simulink model "SAR_model"  (R2022a)
settings: Solver=VariableStepAuto  StartTime=0.0  StopTime=100  FixedStep=5
values from neighbouring files (symbols this model uses):
  C = diag([0.1789, 0.3915,  0.3126, 0.1245])    [Initialization.m]
  delta = 0.5*[ 1.3523 1.2784 2.1553 ... (first row only)    [Initialization.m]
  eta0 = [0 0 0 0]    [Initialization.m]
  J = [10 1 1; 1 8 0; 1 0 6]    [Initialization.m]
  K = diag([2.5514, 5.1806, 3.8173, 6.1966])    [Initialization.m]
  psi0 = delta*transpose(w0)    [Initialization.m]
  q0 = angle2quat(Phi0(1),Phi0(2),Phi0(3))    [Initialization.m]
  qd = angle2quat(Phid(1),Phid(2),Phid(3))    [Initialization.m]
  w0 = [pi/12 pi/24 0]    [Initialization.m]
  wd = [0 0 0]    [Initialization.m]
undefined symbols (not defined in the file or in its folder): deg, magnitude, rad, s
libraries: aerolibconvert2 x3, sharedtransform x2, rllib x2, aerolibutil x1
settings Model: PacingRate=1000  Creator=Ali  LastModifiedBy=Shayan
settings SolverCC: MaxConsecutiveZCs=1  MaxConsecutiveMinStep=10  ZeroCrossAlgorithm=Adaptive  AlgebraicLoopSolver=TrustRegion
settings DataIOCC: SaveFinalState=on  SaveState=on  LoggingToFile=on
settings DebuggingCC: AlgebraicLoopMsg=none  UnconnectedInputMsg=warning  UnconnectedOutputMsg=warning  UnconnectedLineMsg=warning  SFMachineParentedDataDiag=warning
settings ModelReferenceCC: ModelReferenceMinAlgLoopOccurrences=on

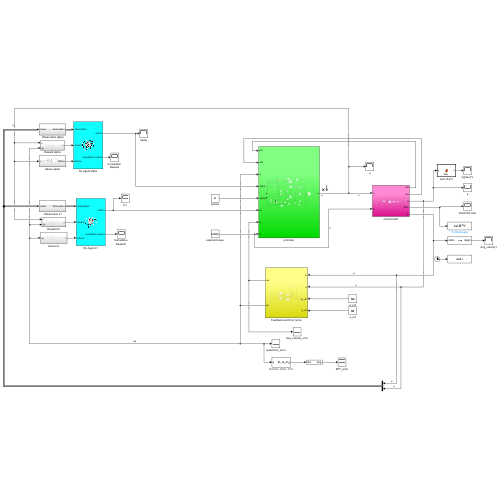
[thumbnail: Simulink's stored preview of the top-level diagram]
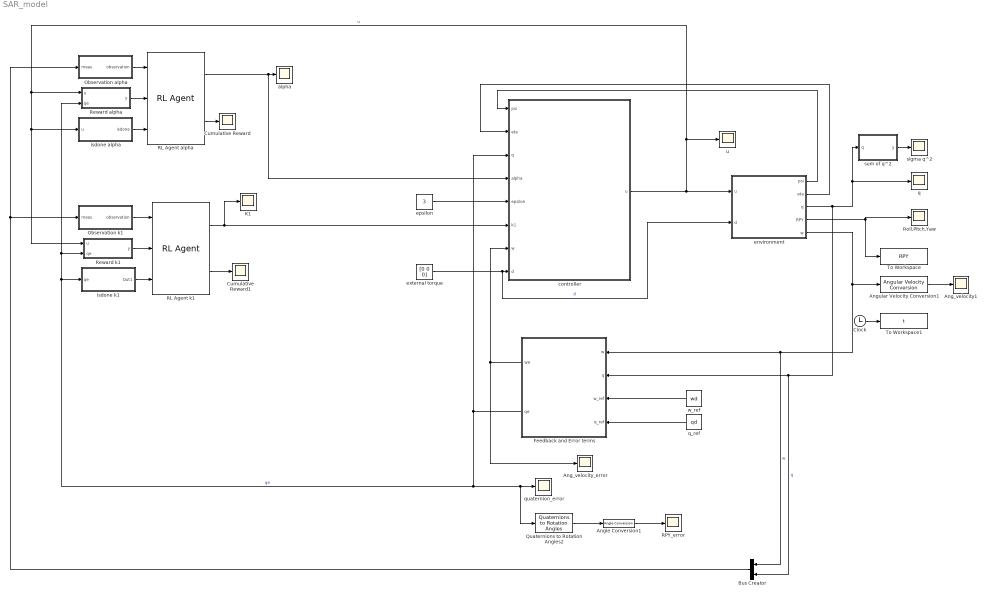
== system SAR_model ==
  " Observation alpha" : Subsystem
  " Observation k1" : Subsystem
  Ang_velocity1 : Scope
  Ang_velocity_error : Scope
  Angle Conversion1 : aerolibconvert2/Angle Conversion  IU=rad  OU=deg
  Angular Velocity Conversion1 : aerolibconvert2/Angular Velocity Conversion  IU=rad/s  OU=deg/s
  Bus Creator : BusCreator  Inputs=2
  Clock : Clock
  Cumulative Reward : Scope
  Cumulative Reward1 : Scope
  Feedback and Error terms : Subsystem
  K1 : Scope
  Quaternions to Rotation Angles2 : sharedtransform/Quaternions to Rotation Angles  rotationOrder=ZYX  aMode=aMode
      settings: SourceProductBaseCode=AE,PW,DR,MT,VE
  RL Agent alpha : rllib/RL Agent  Agent=agent3_Trained  ExternalActionAsInput=off  ProvideLastAction=off  ProvideCumRwd=on  TreatAsDirectFeedthrough=on  UseStrictObservationDataTypes=off
      settings: SourceProductName=Reinforcement Learning
  RL Agent k1 : rllib/RL Agent  Agent=agent1  ExternalActionAsInput=off  ProvideLastAction=off  ProvideCumRwd=on  TreatAsDirectFeedthrough=on  UseStrictObservationDataTypes=off
      settings: SourceProductName=Reinforcement Learning
  RPY_error : Scope
  Reward alpha : Subsystem
  Reward k1 : Subsystem
  Roll,Pitch,Yaw : Scope
  To Workspace : ToWorkspace  VariableName=RPY  SaveFormat=Timeseries
  To Workspace1 : ToWorkspace  VariableName=t  SaveFormat=Timeseries
  alpha : Scope
  "controller " : Subsystem
  environment : Subsystem
  epsilon : Constant  Value=3
  external torque : Constant  Value=[0 0 0]
  isdone alpha : Subsystem
  isdone k1 : Subsystem
  q : Scope
  q_ref : Constant  Value=qd
  quaternion_error : Scope
  sigma q^2 : Scope
  sum of q^2 : MATLAB Function  TreatAsAtomicUnit=on
  u : Scope
  w_ref : Constant  Value=wd
  wires:
  epsilon/1 -> "controller "/5(epsilon)
  external torque/1 -> environment/2(d), "controller "/8(d)  "d"
  Feedback and Error terms/1(we) -> Ang_velocity_error/1, "controller "/7(w)
  w_ref/1 -> Feedback and Error terms/3(w_ref)
  q_ref/1 -> Feedback and Error terms/4(q_ref)
  Quaternions to Rotation Angles2/1 -> Angle Conversion1/1
  Angle Conversion1/1 -> RPY_error/1
  isdone alpha/1(isdone) -> RL Agent alpha/3
  Reward alpha/1(y) -> RL Agent alpha/2
  RL Agent alpha/2 -> Cumulative Reward/1
  " Observation alpha"/1(observation) -> RL Agent alpha/1
  "controller "/1(u) -> environment/1(u), Reward alpha/1(u), isdone alpha/1(u), Reward k1/1(u), u/1  "u"
  RL Agent k1/2 -> Cumulative Reward1/1
  Bus Creator/1 -> " Observation alpha"/1(meas), " Observation k1"/1(meas)
  Reward k1/1(y) -> RL Agent k1/2
  " Observation k1"/1(observation) -> RL Agent k1/1
  Feedback and Error terms/2(qe) -> quaternion_error/1, Quaternions to Rotation Angles2/1, Reward alpha/2(qe), Reward k1/2(qe), isdone k1/1(qe), "controller "/3(q)  "qe"
  RL Agent alpha/1 -> "controller "/4(alpha), alpha/1
  isdone k1/1(Out1) -> RL Agent k1/3
  Clock/1 -> To Workspace1/1
  RL Agent k1/1 -> K1/1, "controller "/6(k1)
  sum of q^2/1(y) -> sigma q^2/1
  environment/3(q) -> sum of q^2/1(q), q/1, Feedback and Error terms/2(q), Bus Creator/2  "q"
  environment/4(RPY) -> To Workspace/1, Roll,Pitch,Yaw/1
  environment/5(w) -> Feedback and Error terms/1(w), Bus Creator/1, Angular Velocity Conversion1/1  "w"
  environment/1(psi) -> "controller "/1(psi)
  environment/2(eta) -> "controller "/2(eta)
  Angular Velocity Conversion1/1 -> Ang_velocity1/1

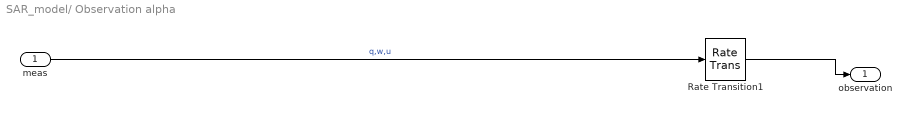
== system SAR_model/ Observation alpha ==
  meas : Inport
  Rate Transition1 : RateTransition
  observation : Outport  VectorParamsAs1DForOutWhenUnconnected=off
  wires:
  meas/1 -> Rate Transition1/1  "q,w,u"
  Rate Transition1/1 -> observation/1

== system SAR_model/ Observation k1 ==
  meas : Inport
  Rate Transition1 : RateTransition
  observation : Outport  VectorParamsAs1DForOutWhenUnconnected=off
  wires:
  meas/1 -> Rate Transition1/1  "q,w,u"
  Rate Transition1/1 -> observation/1

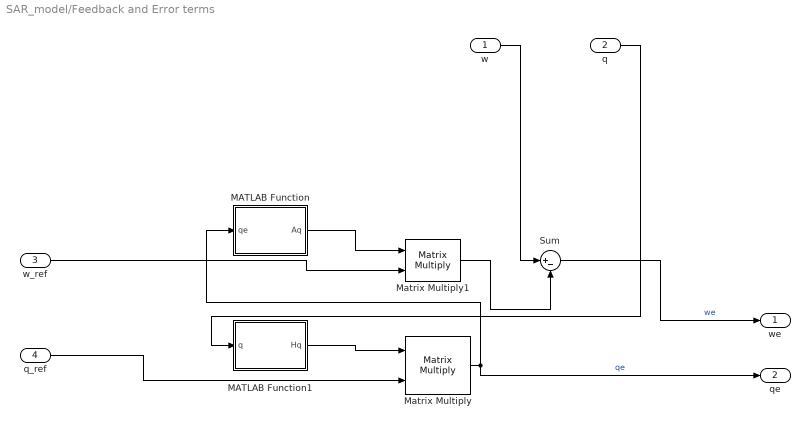
== system SAR_model/Feedback and Error terms ==
  w : Inport
  q : Inport  Port=2
  w_ref : Inport  Port=3
  q_ref : Inport  Port=4
  MATLAB Function : MATLAB Function  TreatAsAtomicUnit=on
  MATLAB Function1 : MATLAB Function  TreatAsAtomicUnit=on
  Matrix Multiply : Product  Multiplication=Matrix(*)
  Matrix Multiply1 : Product  Multiplication=Matrix(*)
  Sum : Sum  Inputs=|+-
  we : Outport
  qe : Outport  Port=2
  wires:
  Sum/1 -> we/1  "we"
  MATLAB Function1/1(Hq) -> Matrix Multiply/1
  Matrix Multiply1/1 -> Sum/2
  Matrix Multiply/1 -> qe/1, MATLAB Function/1(qe)  "qe"
  w/1 -> Sum/1
  q_ref/1 -> Matrix Multiply/2
  q/1 -> MATLAB Function1/1(q)
  w_ref/1 -> Matrix Multiply1/2
  MATLAB Function/1(Aq) -> Matrix Multiply1/1

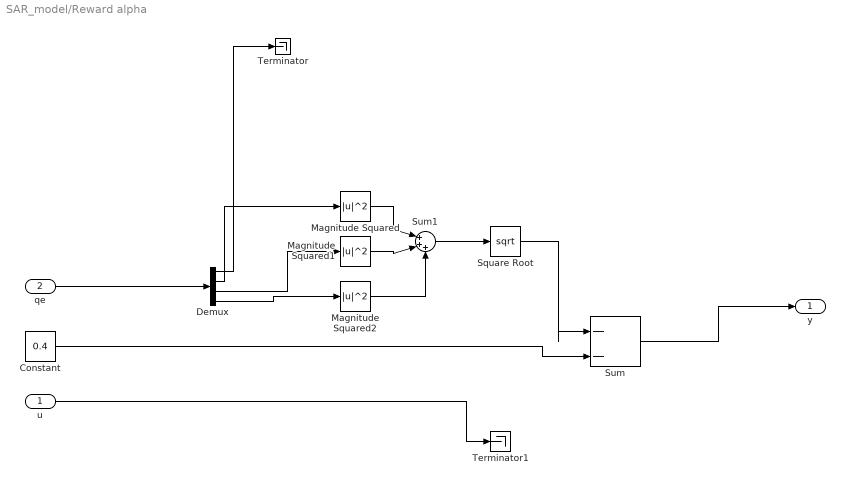
== system SAR_model/Reward alpha ==
  u : Inport
  qe : Inport  Port=2
  Constant : Constant  Value=0.4
  Demux : Demux
  Magnitude Squared : Math  Operator=magnitude^2
  Magnitude Squared1 : Math  Operator=magnitude^2
  Magnitude Squared2 : Math  Operator=magnitude^2
  Square Root : Sqrt
  Sum : Sum  Inputs=|--
  Sum1 : Sum  Inputs=|+++
  Terminator : Terminator
  Terminator1 : Terminator
  y : Outport
  wires:
  u/1 -> Terminator1/1
  Constant/1 -> Sum/2
  Sum/1 -> y/1
  qe/1 -> Demux/1
  Demux/1 -> Terminator/1
  Demux/2 -> Magnitude Squared/1
  Demux/3 -> Magnitude Squared1/1
  Demux/4 -> Magnitude Squared2/1
  Magnitude Squared/1 -> Sum1/1
  Magnitude Squared1/1 -> Sum1/2
  Magnitude Squared2/1 -> Sum1/3
  Sum1/1 -> Square Root/1
  Square Root/1 -> Sum/1

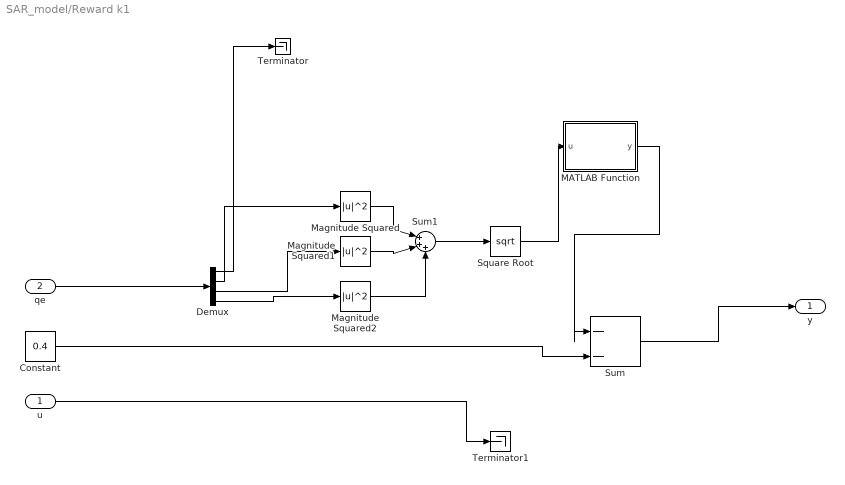
== system SAR_model/Reward k1 ==
  u : Inport
  qe : Inport  Port=2
  Constant : Constant  Value=0.4
  Demux : Demux
  MATLAB Function : MATLAB Function  TreatAsAtomicUnit=on
  Magnitude Squared : Math  Operator=magnitude^2
  Magnitude Squared1 : Math  Operator=magnitude^2
  Magnitude Squared2 : Math  Operator=magnitude^2
  Square Root : Sqrt
  Sum : Sum  Inputs=|--
  Sum1 : Sum  Inputs=|+++
  Terminator : Terminator
  Terminator1 : Terminator
  y : Outport
  wires:
  u/1 -> Terminator1/1
  Constant/1 -> Sum/2
  Sum/1 -> y/1
  qe/1 -> Demux/1
  Demux/1 -> Terminator/1
  Demux/2 -> Magnitude Squared/1
  Demux/3 -> Magnitude Squared1/1
  Demux/4 -> Magnitude Squared2/1
  Magnitude Squared/1 -> Sum1/1
  Magnitude Squared1/1 -> Sum1/2
  Magnitude Squared2/1 -> Sum1/3
  Sum1/1 -> Square Root/1
  Square Root/1 -> MATLAB Function/1(u)
  MATLAB Function/1(y) -> Sum/1

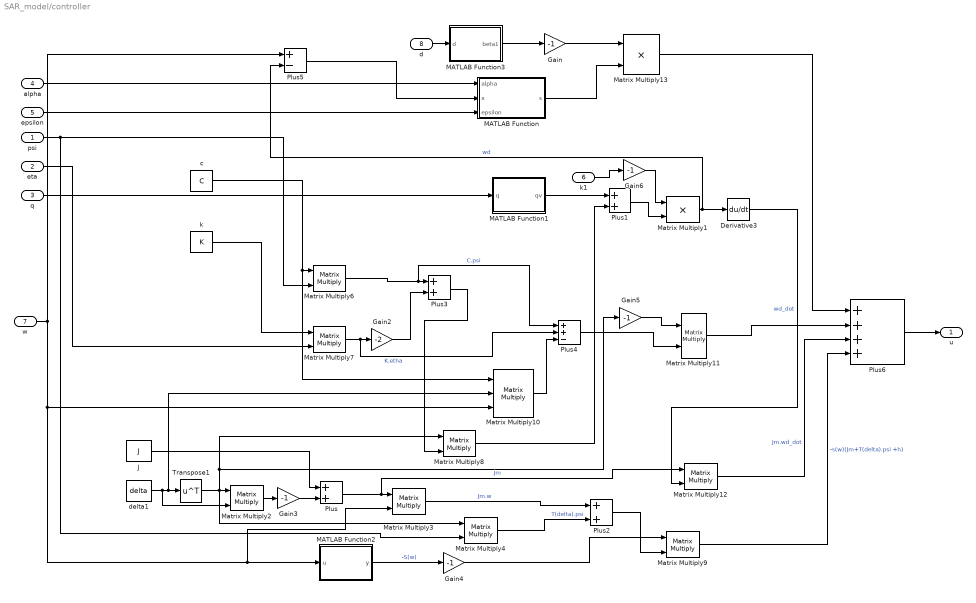
== system SAR_model/controller  ==
  psi : Inport
  eta : Inport  Port=2
  q : Inport  Port=3
  alpha : Inport  Port=4
  epsilon : Inport  Port=5
  k1 : Inport  Port=6
  w : Inport  Port=7
  d : Inport  Port=8
  Derivative3 : Derivative
  Gain{,3..6} (5 alike) : Gain  Gain=-1
  Gain2 : Gain  Gain=-2
  J : Constant  Value=J
  MATLAB Function : MATLAB Function  TreatAsAtomicUnit=on
  MATLAB Function1 : MATLAB Function  TreatAsAtomicUnit=on
  MATLAB Function2 : MATLAB Function  TreatAsAtomicUnit=on
  MATLAB Function3 : MATLAB Function  TreatAsAtomicUnit=on
  Matrix Multiply1 : Product
  Matrix Multiply10 : Product  Inputs=3  Multiplication=Matrix(*)
  Matrix Multiply{2..4,7..9,11..12} (8 alike) : Product  Multiplication=Matrix(*)
  Matrix Multiply13 : Product
  Matrix Multiply6 : Product  Multiplication=Matrix(*)  InputSameDT=on
  Plus{,1..3} (4 alike) : Sum
  Plus4 : Sum  Inputs=++-
  Plus5 : Sum  Inputs=+-
  Plus6 : Sum  Inputs=++++
  Transpose1 : Math  Operator=transpose
  c : Constant  Value=C
  delta1 : Constant  Value=delta
  k : Constant  Value=K
  u : Outport
  wires:
  Matrix Multiply6/1 -> Plus4/1, Plus3/1  "C.psi"
  Matrix Multiply7/1 -> Plus4/2, Gain2/1  "K.etha"
  Gain2/1 -> Plus3/2
  Plus3/1 -> Matrix Multiply8/2
  alpha/1 -> MATLAB Function/1(alpha)
  epsilon/1 -> MATLAB Function/3(epsilon)
  q/1 -> MATLAB Function1/1(q)
  Matrix Multiply8/1 -> Plus1/2
  MATLAB Function1/1(qv) -> Plus1/1
  k1/1 -> Gain6/1
  Matrix Multiply1/1 -> Derivative3/1, Plus5/2  "wd"
  psi/1 -> Matrix Multiply6/2, Matrix Multiply4/2
  eta/1 -> Matrix Multiply7/2
  delta1/1 -> Matrix Multiply2/2, Matrix Multiply10/2, Transpose1/1
  Plus/1 -> Matrix Multiply12/1, Matrix Multiply3/1  "Jm"
  J/1 -> Plus/1
  Gain3/1 -> Plus/2
  Matrix Multiply2/1 -> Gain3/1
  Transpose1/1 -> Matrix Multiply8/1, Gain5/1, Matrix Multiply2/1, Matrix Multiply4/1
  w/1 -> Plus5/1, Matrix Multiply10/3, Matrix Multiply3/2, MATLAB Function2/1(u)
  MATLAB Function2/1(y) -> Gain4/1  "-S(w)"
  Matrix Multiply3/1 -> Plus2/1  "Jm.w"
  Matrix Multiply4/1 -> Plus2/2  "T(delta).psi"
  Plus2/1 -> Matrix Multiply9/2
  Matrix Multiply10/1 -> Plus4/3
  Plus4/1 -> Matrix Multiply11/2
  Gain5/1 -> Matrix Multiply11/1
  d/1 -> MATLAB Function3/1(d)
  Plus5/1 -> MATLAB Function/2(x)
  Matrix Multiply9/1 -> Plus6/4  "-s(w)(Jm+T(delta).psi +h)"
  Matrix Multiply11/1 -> Plus6/2
  Matrix Multiply12/1 -> Plus6/3  "Jm.wd_dot"
  Matrix Multiply13/1 -> Plus6/1
  Plus6/1 -> u/1
  Derivative3/1 -> Matrix Multiply12/2  "wd_dot"
  c/1 -> Matrix Multiply10/1, Matrix Multiply6/1
  k/1 -> Matrix Multiply7/1
  Plus1/1 -> Matrix Multiply1/2
  Gain6/1 -> Matrix Multiply1/1
  MATLAB Function/1(s) -> Matrix Multiply13/2
  MATLAB Function3/1(beta1) -> Gain/1
  Gain/1 -> Matrix Multiply13/1
  Gain4/1 -> Matrix Multiply9/1

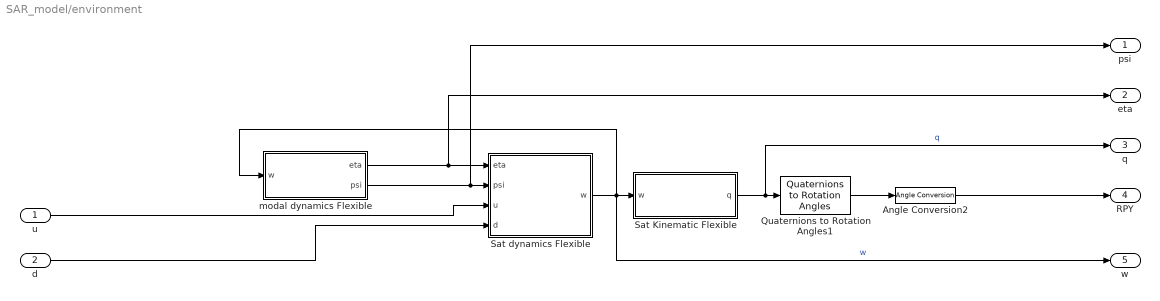
== system SAR_model/environment ==
  u : Inport
  d : Inport  Port=2
  Angle Conversion2 : aerolibconvert2/Angle Conversion  IU=rad  OU=deg
  Quaternions to Rotation Angles1 : sharedtransform/Quaternions to Rotation Angles  rotationOrder=ZYX  aMode=aMode
      settings: SourceProductBaseCode=AE,PW,DR,MT,VE
  Sat Kinematic Flexible : Subsystem
  Sat dynamics Flexible : Subsystem
  modal dynamics Flexible : Subsystem
  psi : Outport
  eta : Outport  Port=2
  q : Outport  Port=3
  RPY : Outport  Port=4
  w : Outport  Port=5
  wires:
  Sat dynamics Flexible/1(w) -> w/1, modal dynamics Flexible/1(w), Sat Kinematic Flexible/1(w)  "w"
  modal dynamics Flexible/1(eta) -> Sat dynamics Flexible/1(eta), eta/1
  modal dynamics Flexible/2(psi) -> Sat dynamics Flexible/2(psi), psi/1
  u/1 -> Sat dynamics Flexible/3(u)
  d/1 -> Sat dynamics Flexible/4(d)
  Sat Kinematic Flexible/1(q) -> q/1, Quaternions to Rotation Angles1/1  "q"
  Quaternions to Rotation Angles1/1 -> Angle Conversion2/1
  Angle Conversion2/1 -> RPY/1

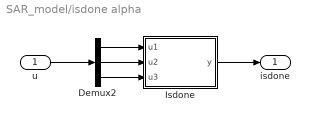
== system SAR_model/isdone alpha ==
  u : Inport
  Demux2 : Demux  Outputs=3
  "Isdone " : MATLAB Function  TreatAsAtomicUnit=on
  isdone : Outport
  wires:
  u/1 -> Demux2/1
  Demux2/1 -> "Isdone "/1(u1)
  Demux2/2 -> "Isdone "/2(u2)
  Demux2/3 -> "Isdone "/3(u3)
  "Isdone "/1(y) -> isdone/1

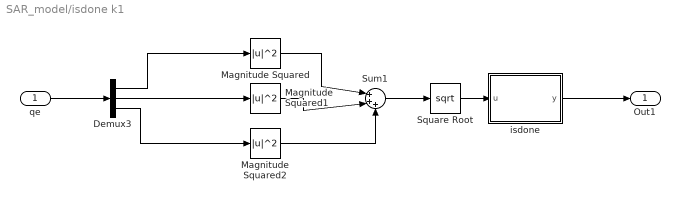
== system SAR_model/isdone k1 ==
  qe : Inport
  Demux3 : Demux  Outputs=3
  Magnitude Squared : Math  Operator=magnitude^2
  Magnitude Squared1 : Math  Operator=magnitude^2
  Magnitude Squared2 : Math  Operator=magnitude^2
  Square Root : Sqrt
  Sum1 : Sum  Inputs=|+++
  isdone : MATLAB Function  TreatAsAtomicUnit=on
  Out1 : Outport
  wires:
  Square Root/1 -> isdone/1(u)
  Magnitude Squared/1 -> Sum1/1
  Demux3/2 -> Magnitude Squared1/1
  Magnitude Squared2/1 -> Sum1/3
  Magnitude Squared1/1 -> Sum1/2
  Demux3/1 -> Magnitude Squared/1
  Sum1/1 -> Square Root/1
  Demux3/3 -> Magnitude Squared2/1
  qe/1 -> Demux3/1
  isdone/1(y) -> Out1/1

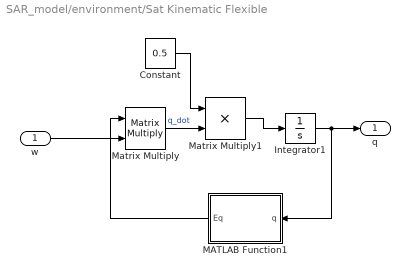
== system SAR_model/environment/Sat Kinematic Flexible ==
  w : Inport
  Constant : Constant  Value=0.5
  Integrator1 : Integrator  InitialCondition=q0  ContinuousStateAttributes='q'
  MATLAB Function1 : MATLAB Function  TreatAsAtomicUnit=on
  Matrix Multiply : Product  Multiplication=Matrix(*)
  Matrix Multiply1 : Product
  q : Outport
  wires:
  Matrix Multiply/1 -> Matrix Multiply1/2  "q_dot"
  w/1 -> Matrix Multiply/2
  Integrator1/1 -> MATLAB Function1/1(q), q/1
  MATLAB Function1/1(Eq) -> Matrix Multiply/1
  Matrix Multiply1/1 -> Integrator1/1
  Constant/1 -> Matrix Multiply1/1

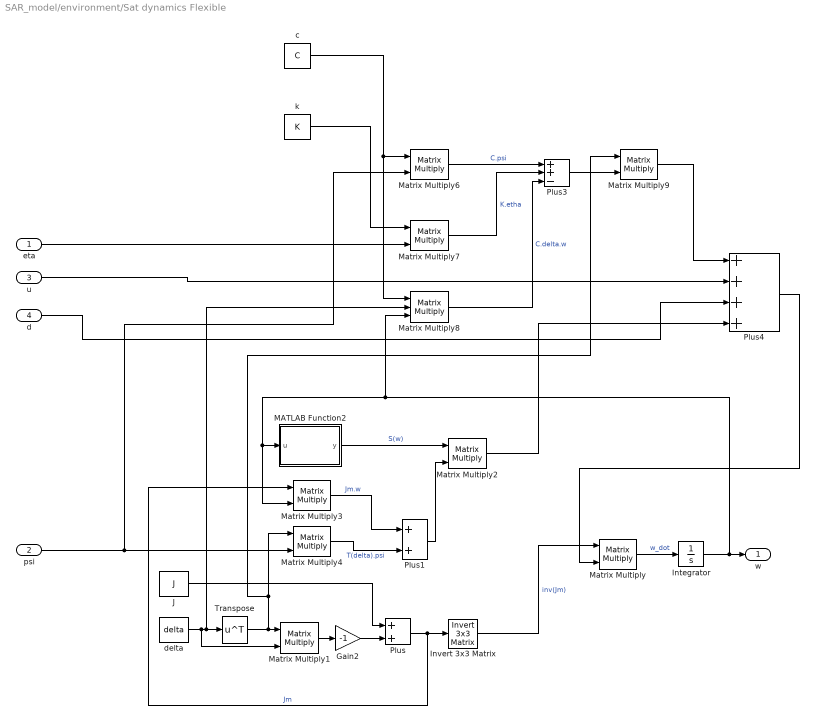
== system SAR_model/environment/Sat dynamics Flexible ==
  eta : Inport
  psi : Inport  Port=2
  u : Inport  Port=3
  d : Inport  Port=4
  Gain2 : Gain  Gain=-1
  Integrator : Integrator  InitialCondition=w0  ContinuousStateAttributes='w'
  Invert 3x3 Matrix : aerolibutil/Invert  3x3 Matrix
  J : Constant  Value=J
  MATLAB Function2 : MATLAB Function  TreatAsAtomicUnit=on
  Matrix Multiply{,1..4,7} (6 alike) : Product  Multiplication=Matrix(*)
  Matrix Multiply6 : Product  Multiplication=Matrix(*)  InputSameDT=on
  Matrix Multiply8 : Product  Inputs=3  Multiplication=Matrix(*)
  Matrix Multiply9 : Product  Multiplication=Matrix(*)  InputSameDT=on
  Plus : Sum
  Plus1 : Sum
  Plus3 : Sum  Inputs=++-
  Plus4 : Sum  Inputs=++++
  Transpose : Math  Operator=transpose
  c : Constant  Value=C  VectorParams1D=off
  delta : Constant  Value=delta
  k : Constant  Value=K  VectorParams1D=off
  w : Outport
  wires:
  Integrator/1 -> Matrix Multiply8/3, Matrix Multiply3/2, MATLAB Function2/1(u), w/1
  delta/1 -> Matrix Multiply1/2, Matrix Multiply8/2, Transpose/1
  Transpose/1 -> Matrix Multiply9/1, Matrix Multiply4/1, Matrix Multiply1/1
  Matrix Multiply1/1 -> Gain2/1
  Gain2/1 -> Plus/2
  J/1 -> Plus/1
  Plus/1 -> Invert 3x3 Matrix/1, Matrix Multiply3/1  "Jm"
  Invert 3x3 Matrix/1 -> Matrix Multiply/1  "inv(Jm)"
  MATLAB Function2/1(y) -> Matrix Multiply2/1  "S(w)"
  psi/1 -> Matrix Multiply6/2, Matrix Multiply4/2
  Matrix Multiply3/1 -> Plus1/1  "Jm.w"
  Matrix Multiply4/1 -> Plus1/2  "T(delta).psi"
  Plus1/1 -> Matrix Multiply2/2
  eta/1 -> Matrix Multiply7/2
  Matrix Multiply6/1 -> Plus3/1  "C.psi"
  Matrix Multiply7/1 -> Plus3/2  "K.etha"
  Matrix Multiply8/1 -> Plus3/3  "C.delta.w"
  Plus3/1 -> Matrix Multiply9/2
  Matrix Multiply9/1 -> Plus4/1
  u/1 -> Plus4/2
  d/1 -> Plus4/3
  Matrix Multiply/1 -> Integrator/1  "w_dot"
  Plus4/1 -> Matrix Multiply/2
  c/1 -> Matrix Multiply8/1, Matrix Multiply6/1
  k/1 -> Matrix Multiply7/1
  Matrix Multiply2/1 -> Plus4/4

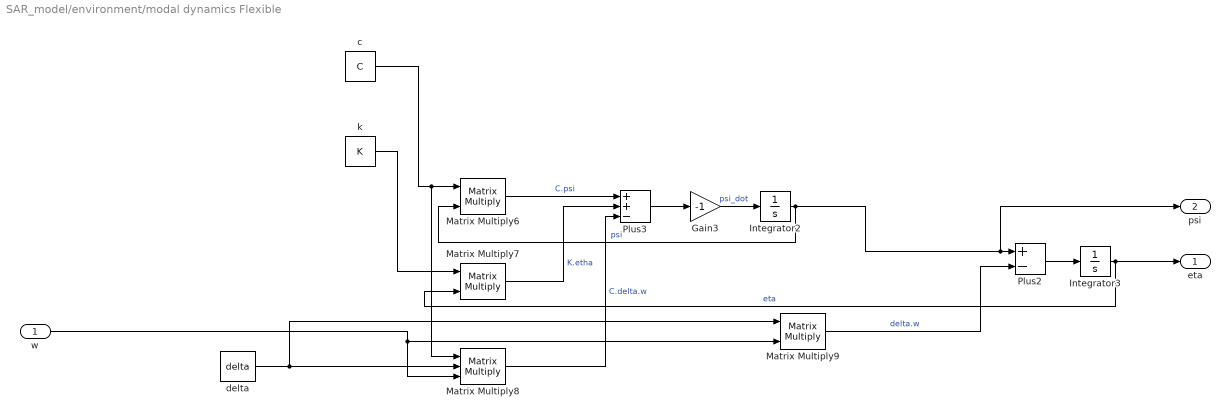
== system SAR_model/environment/modal dynamics Flexible ==
  w : Inport
  Gain3 : Gain  Gain=-1
  Integrator2 : Integrator  InitialCondition=psi0  ContinuousStateAttributes='psi'
  Integrator3 : Integrator  InitialCondition=eta0  ContinuousStateAttributes='eta'
  Matrix Multiply6 : Product  Multiplication=Matrix(*)  InputSameDT=on
  Matrix Multiply7 : Product  Multiplication=Matrix(*)
  Matrix Multiply8 : Product  Inputs=3  Multiplication=Matrix(*)
  Matrix Multiply9 : Product  Multiplication=Matrix(*)
  Plus2 : Sum  Inputs=+-
  Plus3 : Sum  Inputs=++-
  c : Constant  Value=C
  delta : Constant  Value=delta
  k : Constant  Value=K
  eta : Outport
  psi : Outport  Port=2
  wires:
  delta/1 -> Matrix Multiply8/2, Matrix Multiply9/1
  Matrix Multiply6/1 -> Plus3/1  "C.psi"
  Matrix Multiply7/1 -> Plus3/2  "K.etha"
  Matrix Multiply8/1 -> Plus3/3  "C.delta.w"
  Plus3/1 -> Gain3/1
  Gain3/1 -> Integrator2/1  "psi_dot"
  Integrator2/1 -> Matrix Multiply6/2, psi/1, Plus2/1  "psi"
  w/1 -> Matrix Multiply9/2, Matrix Multiply8/3
  Matrix Multiply9/1 -> Plus2/2  "delta.w"
  Plus2/1 -> Integrator3/1
  Integrator3/1 -> Matrix Multiply7/2, eta/1  "eta"
  c/1 -> Matrix Multiply8/1, Matrix Multiply6/1
  k/1 -> Matrix Multiply7/1

== matlab function SAR_model/Feedback and Error terms/MATLAB Function ==
  data: qe input; Aq output
function Aq = fcn(qe)

qe0 = qe(1);
qe1 = qe(2);
qe2 = qe(3);
qe3 = qe(4);


Aq11 = qe1^2-qe2^2-qe3^2+qe0^2;
Aq12 = 2*((qe1*qe2)+(qe3*qe0));
Aq13 = 2*((qe1*qe3)-(qe2*qe0));
Aq21 = 2*((qe1*qe2)-(qe3*qe0));
Aq22 = -qe1^2+qe2^2+qe3^2+qe0^2;
Aq23 = 2*((qe1*qe0)+(qe2*qe3));
Aq31 = 2*((qe1*qe3)+(qe2*qe0));
Aq32 = 2*((qe2*qe3)-(qe1*qe0));
Aq33 = -qe1^2-qe2^2+qe3^2+qe0^2;

Aq = [Aq11 Aq12 Aq13;
      Aq21 Aq22 Aq23;
      Aq31 Aq32 Aq33];

== matlab function SAR_model/sum of q^2 ==
  data: q input; y output
function y = fcn(q)

y = q(1)^2+q(2)^2+q(3)^2+q(4)^2;

== matlab function SAR_model/Feedback and Error terms/MATLAB Function1 ==
  data: q input; Hq output
function Hq = fcn(q)


Hq=[q(1) q(2) q(3) q(4);
    -q(2) q(1) q(4) -q(3);
    -q(3) -q(4) q(1) q(2); 
    -q(4) q(3) -q(2) q(1)];

== matlab function SAR_model/controller /MATLAB Function ==
  data: alpha input; s output; x input; epsilon input
function s = fcn(alpha,x,epsilon)
z=zeros(1,length(x));
for i=1:length(x)
if abs(x(i))>epsilon
    z(i)=x(i);
elseif abs(x(i))<=epsilon
    z(i)=((sign(x(i)))*(abs(x(i)))^alpha)/epsilon^(alpha-1);
end
end
s=z';

== matlab function SAR_model/controller /MATLAB Function1 ==
  data: q input; qv output
function qv = fcn(q)
x=zeros(1,3);
x(1)=q(2);
x(2)=q(3);
x(3)=q(4);
qv=x';

== matlab function SAR_model/controller /MATLAB Function2 ==
  data: u input; y output
function y = fcn(u)
w1 = u(1);
w2 = u(2);
w3 = u(3);
y = [ 0 w3 -w2;
      -w3 0 w1;
      w2 -w1 0];

== matlab function SAR_model/controller /MATLAB Function3 ==
  data: d input; beta1 output
function beta1 = fcn(d)


beta1 = max(norm(d), 14)+1;

== matlab function SAR_model/environment/Sat Kinematic Flexible/MATLAB Function1 ==
  data: q input; Eq output
function Eq = fcn(q)
q1 = q(1);
q2 = q(2);
q3= q(3);
q4 = q(4);

Eq = [ -q2 -q3 -q4 ;
           q1 -q4  q3;
           q4 q1 -q2;
           -q3 q2 q1];

== matlab function SAR_model/Reward k1/MATLAB Function ==
  data: u input; y output
function y = fcn(u)

y = sqrt((1.4*1e-5-u)^2)

== matlab function SAR_model/isdone k1/isdone ==
  data: u input; y output
function y = fcn(u)

if  u<=(1.4*1e-5)
    y=1;
else
    y=0;
end

== matlab function SAR_model/isdone alpha/Isdone  ==
  data: u1 input; y output; u2 input; u3 input
function y = fcn(u1,u2,u3)
if u1>1000 && u2>1000
    y=1;
elseif u1>1000 && u3>1000
    y=1;
elseif u2>1000 && u3>1000
    y=1;
else
    y=0;
end
end

== matlab function SAR_model/environment/Sat dynamics Flexible/MATLAB Function2 ==
  data: u input; y output
function y = fcn(u)
w1 = u(1);
w2 = u(2);
w3 = u(3);
y = [ 0 w3 -w2;
      -w3 0 w1;
      w2 -w1 0];
